simulink model "GS_model"  (R2018b)
settings: Solver=ode5  StartTime=0.0  StopTime=SimuStopTime  FixedStep=T_Simu  RelTol=1e-3
InitFcn:
  | Initial
undefined symbols (not defined in the file or in its folder): Aba10, Aba20, aeroCIP2006_S, aeroCIP2006_X, aeroCIP2006_Y, Agl0, Ass_kS, Ass_n1, Ass_n2, Ass_n3, Ass_n4, Ass_Noise, Ass_R, Ass_Resolution, Ass_TmOrder, AssA_Fix_Abs, AssB_Fix_Abs, AssC_Fix_Abs, AssD_Fix_Abs, AssE_Fix_Aps, AssF_Fix_Aps, C, c_max, c_min, Cd, CenterOfFigNX, CenterOfFigNY, CenterOfFigNZ, CenterOfFigP1, CenterOfFigP2, CenterOfFigPX, CenterOfFigPY, CenterOfFigPZ, Cmu, Crou, DEG2RAD, DiscIntNeverNeededParam, Eg_Dir, Eg_F, Eg_PrepareTime, Eg_r_L_L, Fw_Abf, Fw_Hmax, Fw_J, Fw_Spd0, Fw_Tmax, git_hash_BaseLine, git_hash_Project, Gnss_Noise_Pos, Gnss_Noise_Vel, Gnss_PropgationTime, GyroA_Fix_Abg, GyroA_Noise, GyroB_Fix_Abg, GyroB_Noise, GyroC_Fix_Abg, GyroC_Noise, GyroD_Fix_Abg, GyroD_Noise, h ... (+94)
libraries: simulink x308, sharedutil x46, aerolibutil x37, sharedtransform x31, vrlib x14, aerolibgravity2 x2
(part 12 of 20)

== system GS_model/Subsystem2/Subsystem/Sensor/Gyro/GyroBModel/GyroErrSet/GyroErrSet ==
  Wgi : Inport
  TC_GyroErrSet_Constant : Inport  Port=2
  TC_GyroErrSet_WildValue : Inport  Port=3
  TC_GyroErrSet_Jump : Inport  Port=4
  TC_StErrSet_Wave : Inport  Port=5
  GyroErrSet_Constant : Subsystem
  GyroErrSet_Jump : Subsystem
  GyroErrSet_Wave : Subsystem
  GyroErrSet_WildValue : Subsystem
  Wgi_g : Outport
  wires:
  GyroErrSet_WildValue/1(w_out) -> GyroErrSet_Jump/1(w_in)
  GyroErrSet_Constant/1(w_out) -> GyroErrSet_WildValue/1(w_in)
  GyroErrSet_Jump/1(w_out) -> GyroErrSet_Wave/1(w_in)
  Wgi/1 -> GyroErrSet_Constant/1(w_in)
  TC_GyroErrSet_Constant/1 -> GyroErrSet_Constant/2(ErrSwitch)
  TC_GyroErrSet_WildValue/1 -> GyroErrSet_WildValue/2(ErrSwitch)
  TC_GyroErrSet_Jump/1 -> GyroErrSet_Jump/2(ErrSet)
  TC_StErrSet_Wave/1 -> GyroErrSet_Wave/2(ErrSet)
  GyroErrSet_Wave/1(w_out) -> Wgi_g/1

== system GS_model/Subsystem2/Subsystem/Sensor/Gyro/GyroBModel/GyroErrSet/If Action Subsystem3 ==
  In1 : Inport
  Action Port : ActionPort  ActionType=else
  Out1 : Outport
  wires:
  In1/1 -> Out1/1

== system GS_model/Subsystem2/Subsystem/Sensor/Gyro/GyroBModel/GyroErrSet/If Action Subsystem4 ==
  In1 : Inport
  Action Port : ActionPort  ActionType=then
  Gain : Gain  Gain=DEG2RAD
  Out1 : Outport
  wires:
  In1/1 -> Gain/1
  Gain/1 -> Out1/1

== system GS_model/Subsystem2/Subsystem/Sensor/Gyro/GyroBModel/GyroErrSet/Triggered Subsystem5 ==
  In1 : Inport
  Enable : EnablePort
  Out1 : Outport  InitialOutput=0
  wires:
  In1/1 -> Out1/1

== system GS_model/Subsystem2/Subsystem/Sensor/Gyro/GyroBModel/GyroErrSet/Triggered Subsystem6 ==
  In1 : Inport
  Enable : EnablePort
  Out1 : Outport  InitialOutput=0
  wires:
  In1/1 -> Out1/1

== system GS_model/Subsystem2/Subsystem/Sensor/Gyro/GyroBModel/GyroErrSet/Triggered Subsystem7 ==
  In1 : Inport
  Enable : EnablePort
  Out1 : Outport
  wires:
  In1/1 -> Out1/1

== system GS_model/Subsystem2/Subsystem/Sensor/Gyro/GyroBModel/GyroErrSet/Triggered Subsystem8 ==
  In1 : Inport
  Enable : EnablePort
  Out1 : Outport
  wires:
  In1/1 -> Out1/1

== system GS_model/Subsystem2/Subsystem/Sensor/Gyro/GyroBModel/GyroErrSet/Triggered Subsystem9 ==
  In1 : Inport
  Enable : EnablePort
  Out1 : Outport
  wires:
  In1/1 -> Out1/1

== system GS_model/Subsystem2/Subsystem/Sensor/Gyro/GyroBModel/GyroMathModel/Triggered Subsystem1 ==
  In1 : Inport
  Enable : EnablePort
  Out1 : Outport  InitialOutput=0
  wires:
  In1/1 -> Out1/1

== system GS_model/Subsystem2/Subsystem/Sensor/Gyro/GyroCModel/GyroErrSet/GyroErrSet ==
  Wgi : Inport
  TC_GyroErrSet_Constant : Inport  Port=2
  TC_GyroErrSet_WildValue : Inport  Port=3
  TC_GyroErrSet_Jump : Inport  Port=4
  TC_StErrSet_Wave : Inport  Port=5
  GyroErrSet_Constant : Subsystem
  GyroErrSet_Jump : Subsystem
  GyroErrSet_Wave : Subsystem
  GyroErrSet_WildValue : Subsystem
  Wgi_g : Outport
  wires:
  GyroErrSet_WildValue/1(w_out) -> GyroErrSet_Jump/1(w_in)
  GyroErrSet_Constant/1(w_out) -> GyroErrSet_WildValue/1(w_in)
  GyroErrSet_Jump/1(w_out) -> GyroErrSet_Wave/1(w_in)
  Wgi/1 -> GyroErrSet_Constant/1(w_in)
  TC_GyroErrSet_Constant/1 -> GyroErrSet_Constant/2(ErrSwitch)
  TC_GyroErrSet_WildValue/1 -> GyroErrSet_WildValue/2(ErrSwitch)
  TC_GyroErrSet_Jump/1 -> GyroErrSet_Jump/2(ErrSet)
  TC_StErrSet_Wave/1 -> GyroErrSet_Wave/2(ErrSet)
  GyroErrSet_Wave/1(w_out) -> Wgi_g/1

== system GS_model/Subsystem2/Subsystem/Sensor/Gyro/GyroCModel/GyroErrSet/If Action Subsystem3 ==
  In1 : Inport
  Action Port : ActionPort  ActionType=else
  Out1 : Outport
  wires:
  In1/1 -> Out1/1

== system GS_model/Subsystem2/Subsystem/Sensor/Gyro/GyroCModel/GyroErrSet/If Action Subsystem4 ==
  In1 : Inport
  Action Port : ActionPort  ActionType=then
  Gain : Gain  Gain=DEG2RAD
  Out1 : Outport
  wires:
  In1/1 -> Gain/1
  Gain/1 -> Out1/1

== system GS_model/Subsystem2/Subsystem/Sensor/Gyro/GyroCModel/GyroErrSet/Triggered Subsystem5 ==
  In1 : Inport
  Enable : EnablePort
  Out1 : Outport  InitialOutput=0
  wires:
  In1/1 -> Out1/1

== system GS_model/Subsystem2/Subsystem/Sensor/Gyro/GyroCModel/GyroErrSet/Triggered Subsystem6 ==
  In1 : Inport
  Enable : EnablePort
  Out1 : Outport  InitialOutput=0
  wires:
  In1/1 -> Out1/1

== system GS_model/Subsystem2/Subsystem/Sensor/Gyro/GyroCModel/GyroErrSet/Triggered Subsystem7 ==
  In1 : Inport
  Enable : EnablePort
  Out1 : Outport
  wires:
  In1/1 -> Out1/1

== system GS_model/Subsystem2/Subsystem/Sensor/Gyro/GyroCModel/GyroErrSet/Triggered Subsystem8 ==
  In1 : Inport
  Enable : EnablePort
  Out1 : Outport
  wires:
  In1/1 -> Out1/1

== system GS_model/Subsystem2/Subsystem/Sensor/Gyro/GyroCModel/GyroErrSet/Triggered Subsystem9 ==
  In1 : Inport
  Enable : EnablePort
  Out1 : Outport
  wires:
  In1/1 -> Out1/1

== system GS_model/Subsystem2/Subsystem/Sensor/Gyro/GyroCModel/GyroMathModel/Triggered Subsystem1 ==
  In1 : Inport
  Enable : EnablePort
  Out1 : Outport  InitialOutput=0
  wires:
  In1/1 -> Out1/1

== system GS_model/Subsystem2/Subsystem/Sensor/Gyro/GyroDModel/GyroErrSet/GyroErrSet ==
  Wgi : Inport
  TC_GyroErrSet_Constant : Inport  Port=2
  TC_GyroErrSet_WildValue : Inport  Port=3
  TC_GyroErrSet_Jump : Inport  Port=4
  TC_StErrSet_Wave : Inport  Port=5
  GyroErrSet_Constant : Subsystem
  GyroErrSet_Jump : Subsystem
  GyroErrSet_Wave : Subsystem
  GyroErrSet_WildValue : Subsystem
  Wgi_g : Outport
  wires:
  GyroErrSet_WildValue/1(w_out) -> GyroErrSet_Jump/1(w_in)
  GyroErrSet_Constant/1(w_out) -> GyroErrSet_WildValue/1(w_in)
  GyroErrSet_Jump/1(w_out) -> GyroErrSet_Wave/1(w_in)
  Wgi/1 -> GyroErrSet_Constant/1(w_in)
  TC_GyroErrSet_Constant/1 -> GyroErrSet_Constant/2(ErrSwitch)
  TC_GyroErrSet_WildValue/1 -> GyroErrSet_WildValue/2(ErrSwitch)
  TC_GyroErrSet_Jump/1 -> GyroErrSet_Jump/2(ErrSet)
  TC_StErrSet_Wave/1 -> GyroErrSet_Wave/2(ErrSet)
  GyroErrSet_Wave/1(w_out) -> Wgi_g/1

== system GS_model/Subsystem2/Subsystem/Sensor/Gyro/GyroDModel/GyroErrSet/If Action Subsystem3 ==
  In1 : Inport
  Action Port : ActionPort  ActionType=else
  Out1 : Outport
  wires:
  In1/1 -> Out1/1

== system GS_model/Subsystem2/Subsystem/Sensor/Gyro/GyroDModel/GyroErrSet/If Action Subsystem4 ==
  In1 : Inport
  Action Port : ActionPort  ActionType=then
  Gain : Gain  Gain=DEG2RAD
  Out1 : Outport
  wires:
  In1/1 -> Gain/1
  Gain/1 -> Out1/1

== system GS_model/Subsystem2/Subsystem/Sensor/Gyro/GyroDModel/GyroErrSet/Triggered Subsystem5 ==
  In1 : Inport
  Enable : EnablePort
  Out1 : Outport  InitialOutput=0
  wires:
  In1/1 -> Out1/1

== system GS_model/Subsystem2/Subsystem/Sensor/Gyro/GyroDModel/GyroErrSet/Triggered Subsystem6 ==
  In1 : Inport
  Enable : EnablePort
  Out1 : Outport  InitialOutput=0
  wires:
  In1/1 -> Out1/1

== system GS_model/Subsystem2/Subsystem/Sensor/Gyro/GyroDModel/GyroErrSet/Triggered Subsystem7 ==
  In1 : Inport
  Enable : EnablePort
  Out1 : Outport
  wires:
  In1/1 -> Out1/1

== system GS_model/Subsystem2/Subsystem/Sensor/Gyro/GyroDModel/GyroErrSet/Triggered Subsystem8 ==
  In1 : Inport
  Enable : EnablePort
  Out1 : Outport
  wires:
  In1/1 -> Out1/1

== system GS_model/Subsystem2/Subsystem/Sensor/Gyro/GyroDModel/GyroErrSet/Triggered Subsystem9 ==
  In1 : Inport
  Enable : EnablePort
  Out1 : Outport
  wires:
  In1/1 -> Out1/1

== system GS_model/Subsystem2/Subsystem/Sensor/Gyro/GyroDModel/GyroMathModel/Triggered Subsystem1 ==
  In1 : Inport
  Enable : EnablePort
  Out1 : Outport  InitialOutput=0
  wires:
  In1/1 -> Out1/1

== system GS_model/Subsystem2/Subsystem/Sensor/Magnetometer/MmModel1/Mm_ErrSet/If Action Subsystem3 ==
  In1 : Inport
  Action Port : ActionPort  ActionType=else
  Out1 : Outport
  wires:
  In1/1 -> Out1/1

== system GS_model/Subsystem2/Subsystem/Sensor/Magnetometer/MmModel1/Mm_ErrSet/If Action Subsystem4 ==
  In1 : Inport
  Action Port : ActionPort  ActionType=then
  Out1 : Outport
  wires:
  In1/1 -> Out1/1

== system GS_model/Subsystem2/Subsystem/Sensor/Magnetometer/MmModel1/Mm_ErrSet/MmErrSet ==
  Mm_MagneticIntensity : Inport
  TC_MmErrSet_Constant : Inport  Port=2
  TC_MmErrSet_Jump : Inport  Port=3
  TC_MmErrSet_Wave : Inport  Port=4
  TC_MmErrSet_WildValue : Inport  Port=5
  MmErrSet_Constant : Subsystem
  MmErrSet_Jump : Subsystem
  MmErrSet_Wave : Subsystem
  MmErrSet_WildValue : Subsystem
  Mm_out : Outport
  wires:
  MmErrSet_WildValue/1(Mm_out) -> MmErrSet_Jump/1(Mm_in)
  MmErrSet_Constant/1(Mm_out) -> MmErrSet_WildValue/1(Mm_in)
  MmErrSet_Jump/1(Mm_out) -> MmErrSet_Wave/1(Mm_in)
  Mm_MagneticIntensity/1 -> MmErrSet_Constant/1(Mm_in)
  TC_MmErrSet_Constant/1 -> MmErrSet_Constant/2(ErrSwitch)
  TC_MmErrSet_WildValue/1 -> MmErrSet_WildValue/2(ErrSwitch)
  TC_MmErrSet_Jump/1 -> MmErrSet_Jump/2(ErrSet)
  TC_MmErrSet_Wave/1 -> MmErrSet_Wave/2(ErrSet)
  MmErrSet_Wave/1(Mm_out) -> Mm_out/1

== system GS_model/Subsystem2/Subsystem/Sensor/Magnetometer/MmModel1/Mm_ErrSet/Triggered Subsystem5 ==
  In1 : Inport
  Enable : EnablePort
  Out1 : Outport  InitialOutput=0
  wires:
  In1/1 -> Out1/1

== system GS_model/Subsystem2/Subsystem/Sensor/Magnetometer/MmModel1/Mm_ErrSet/Triggered Subsystem6 ==
  In1 : Inport
  Enable : EnablePort
  Out1 : Outport  InitialOutput=0
  wires:
  In1/1 -> Out1/1

== system GS_model/Subsystem2/Subsystem/Sensor/Magnetometer/MmModel1/Mm_ErrSet/Triggered Subsystem7 ==
  In1 : Inport
  Enable : EnablePort
  Out1 : Outport
  wires:
  In1/1 -> Out1/1

== system GS_model/Subsystem2/Subsystem/Sensor/Magnetometer/MmModel1/Mm_ErrSet/Triggered Subsystem8 ==
  In1 : Inport
  Enable : EnablePort
  Out1 : Outport
  wires:
  In1/1 -> Out1/1

== system GS_model/Subsystem2/Subsystem/Sensor/Magnetometer/MmModel1/Mm_ErrSet/Triggered Subsystem9 ==
  In1 : Inport
  Enable : EnablePort
  Out1 : Outport
  wires:
  In1/1 -> Out1/1

== system GS_model/Subsystem2/Subsystem/Sensor/Magnetometer/MmModel2/Mm_ErrSet/If Action Subsystem3 ==
  In1 : Inport
  Action Port : ActionPort  ActionType=else
  Out1 : Outport
  wires:
  In1/1 -> Out1/1

== system GS_model/Subsystem2/Subsystem/Sensor/Magnetometer/MmModel2/Mm_ErrSet/If Action Subsystem4 ==
  In1 : Inport
  Action Port : ActionPort  ActionType=then
  Out1 : Outport
  wires:
  In1/1 -> Out1/1

== system GS_model/Subsystem2/Subsystem/Sensor/Magnetometer/MmModel2/Mm_ErrSet/MmErrSet ==
  Mm_MagneticIntensity : Inport
  TC_MmErrSet_Constant : Inport  Port=2
  TC_MmErrSet_Jump : Inport  Port=3
  TC_MmErrSet_Wave : Inport  Port=4
  TC_MmErrSet_WildValue : Inport  Port=5
  MmErrSet_Constant : Subsystem
  MmErrSet_Jump : Subsystem
  MmErrSet_Wave : Subsystem
  MmErrSet_WildValue : Subsystem
  Mm_out : Outport
  wires:
  MmErrSet_Wave/1(Mm_out) -> Mm_out/1
  TC_MmErrSet_Wave/1 -> MmErrSet_Wave/2(ErrSet)
  TC_MmErrSet_Jump/1 -> MmErrSet_Jump/2(ErrSet)
  TC_MmErrSet_WildValue/1 -> MmErrSet_WildValue/2(ErrSwitch)
  TC_MmErrSet_Constant/1 -> MmErrSet_Constant/2(ErrSwitch)
  Mm_MagneticIntensity/1 -> MmErrSet_Constant/1(Mm_in)
  MmErrSet_Jump/1(Mm_out) -> MmErrSet_Wave/1(Mm_in)
  MmErrSet_Constant/1(Mm_out) -> MmErrSet_WildValue/1(Mm_in)
  MmErrSet_WildValue/1(Mm_out) -> MmErrSet_Jump/1(Mm_in)

== system GS_model/Subsystem2/Subsystem/Sensor/Magnetometer/MmModel2/Mm_ErrSet/Triggered Subsystem5 ==
  In1 : Inport
  Enable : EnablePort
  Out1 : Outport  InitialOutput=0
  wires:
  In1/1 -> Out1/1

== system GS_model/Subsystem2/Subsystem/Sensor/Magnetometer/MmModel2/Mm_ErrSet/Triggered Subsystem6 ==
  In1 : Inport
  Enable : EnablePort
  Out1 : Outport  InitialOutput=0
  wires:
  In1/1 -> Out1/1

== system GS_model/Subsystem2/Subsystem/Sensor/Magnetometer/MmModel2/Mm_ErrSet/Triggered Subsystem7 ==
  In1 : Inport
  Enable : EnablePort
  Out1 : Outport
  wires:
  In1/1 -> Out1/1

== system GS_model/Subsystem2/Subsystem/Sensor/Magnetometer/MmModel2/Mm_ErrSet/Triggered Subsystem8 ==
  In1 : Inport
  Enable : EnablePort
  Out1 : Outport
  wires:
  In1/1 -> Out1/1

== system GS_model/Subsystem2/Subsystem/Sensor/Magnetometer/MmModel2/Mm_ErrSet/Triggered Subsystem9 ==
  In1 : Inport
  Enable : EnablePort
  Out1 : Outport
  wires:
  In1/1 -> Out1/1

== system GS_model/Subsystem2/Subsystem/Sensor/Magnetometer/MmModel3/Mm_ErrSet/If Action Subsystem3 ==
  In1 : Inport
  Action Port : ActionPort  ActionType=else
  Out1 : Outport
  wires:
  In1/1 -> Out1/1

== system GS_model/Subsystem2/Subsystem/Sensor/Magnetometer/MmModel3/Mm_ErrSet/If Action Subsystem4 ==
  In1 : Inport
  Action Port : ActionPort  ActionType=then
  Out1 : Outport
  wires:
  In1/1 -> Out1/1

== system GS_model/Subsystem2/Subsystem/Sensor/Magnetometer/MmModel3/Mm_ErrSet/MmErrSet ==
  Mm_MagneticIntensity : Inport
  TC_MmErrSet_Constant : Inport  Port=2
  TC_MmErrSet_Jump : Inport  Port=3
  TC_MmErrSet_Wave : Inport  Port=4
  TC_MmErrSet_WildValue : Inport  Port=5
  MmErrSet_Constant : Subsystem
  MmErrSet_Jump : Subsystem
  MmErrSet_Wave : Subsystem
  MmErrSet_WildValue : Subsystem
  Mm_out : Outport
  wires:
  MmErrSet_WildValue/1(Mm_out) -> MmErrSet_Jump/1(Mm_in)
  MmErrSet_Constant/1(Mm_out) -> MmErrSet_WildValue/1(Mm_in)
  MmErrSet_Jump/1(Mm_out) -> MmErrSet_Wave/1(Mm_in)
  Mm_MagneticIntensity/1 -> MmErrSet_Constant/1(Mm_in)
  TC_MmErrSet_Constant/1 -> MmErrSet_Constant/2(ErrSwitch)
  TC_MmErrSet_WildValue/1 -> MmErrSet_WildValue/2(ErrSwitch)
  TC_MmErrSet_Jump/1 -> MmErrSet_Jump/2(ErrSet)
  TC_MmErrSet_Wave/1 -> MmErrSet_Wave/2(ErrSet)
  MmErrSet_Wave/1(Mm_out) -> Mm_out/1

== system GS_model/Subsystem2/Subsystem/Sensor/Magnetometer/MmModel3/Mm_ErrSet/Triggered Subsystem5 ==
  In1 : Inport
  Enable : EnablePort
  Out1 : Outport  InitialOutput=0
  wires:
  In1/1 -> Out1/1

== system GS_model/Subsystem2/Subsystem/Sensor/Magnetometer/MmModel3/Mm_ErrSet/Triggered Subsystem6 ==
  In1 : Inport
  Enable : EnablePort
  Out1 : Outport  InitialOutput=0
  wires:
  In1/1 -> Out1/1

== system GS_model/Subsystem2/Subsystem/Sensor/Magnetometer/MmModel3/Mm_ErrSet/Triggered Subsystem7 ==
  In1 : Inport
  Enable : EnablePort
  Out1 : Outport
  wires:
  In1/1 -> Out1/1

== system GS_model/Subsystem2/Subsystem/Sensor/Magnetometer/MmModel3/Mm_ErrSet/Triggered Subsystem8 ==
  In1 : Inport
  Enable : EnablePort
  Out1 : Outport
  wires:
  In1/1 -> Out1/1

== system GS_model/Subsystem2/Subsystem/Sensor/Magnetometer/MmModel3/Mm_ErrSet/Triggered Subsystem9 ==
  In1 : Inport
  Enable : EnablePort
  Out1 : Outport
  wires:
  In1/1 -> Out1/1

== system GS_model/Subsystem2/Subsystem/Sensor/Magnetometer/MmModel4/Mm_ErrSet/If Action Subsystem3 ==
  In1 : Inport
  Action Port : ActionPort  ActionType=else
  Out1 : Outport
  wires:
  In1/1 -> Out1/1

== system GS_model/Subsystem2/Subsystem/Sensor/Magnetometer/MmModel4/Mm_ErrSet/If Action Subsystem4 ==
  In1 : Inport
  Action Port : ActionPort  ActionType=then
  Out1 : Outport
  wires:
  In1/1 -> Out1/1

== system GS_model/Subsystem2/Subsystem/Sensor/Magnetometer/MmModel4/Mm_ErrSet/MmErrSet ==
  Mm_MagneticIntensity : Inport
  TC_MmErrSet_Constant : Inport  Port=2
  TC_MmErrSet_Jump : Inport  Port=3
  TC_MmErrSet_Wave : Inport  Port=4
  TC_MmErrSet_WildValue : Inport  Port=5
  MmErrSet_Constant : Subsystem
  MmErrSet_Jump : Subsystem
  MmErrSet_Wave : Subsystem
  MmErrSet_WildValue : Subsystem
  Mm_out : Outport
  wires:
  MmErrSet_Wave/1(Mm_out) -> Mm_out/1
  TC_MmErrSet_Wave/1 -> MmErrSet_Wave/2(ErrSet)
  TC_MmErrSet_Jump/1 -> MmErrSet_Jump/2(ErrSet)
  TC_MmErrSet_WildValue/1 -> MmErrSet_WildValue/2(ErrSwitch)
  TC_MmErrSet_Constant/1 -> MmErrSet_Constant/2(ErrSwitch)
  Mm_MagneticIntensity/1 -> MmErrSet_Constant/1(Mm_in)
  MmErrSet_Jump/1(Mm_out) -> MmErrSet_Wave/1(Mm_in)
  MmErrSet_Constant/1(Mm_out) -> MmErrSet_WildValue/1(Mm_in)
  MmErrSet_WildValue/1(Mm_out) -> MmErrSet_Jump/1(Mm_in)

== system GS_model/Subsystem2/Subsystem/Sensor/Magnetometer/MmModel4/Mm_ErrSet/Triggered Subsystem5 ==
  In1 : Inport
  Enable : EnablePort
  Out1 : Outport  InitialOutput=0
  wires:
  In1/1 -> Out1/1

== system GS_model/Subsystem2/Subsystem/Sensor/Magnetometer/MmModel4/Mm_ErrSet/Triggered Subsystem6 ==
  In1 : Inport
  Enable : EnablePort
  Out1 : Outport  InitialOutput=0
  wires:
  In1/1 -> Out1/1

== system GS_model/Subsystem2/Subsystem/Sensor/Magnetometer/MmModel4/Mm_ErrSet/Triggered Subsystem7 ==
  In1 : Inport
  Enable : EnablePort
  Out1 : Outport
  wires:
  In1/1 -> Out1/1

== system GS_model/Subsystem2/Subsystem/Sensor/Magnetometer/MmModel4/Mm_ErrSet/Triggered Subsystem8 ==
  In1 : Inport
  Enable : EnablePort
  Out1 : Outport
  wires:
  In1/1 -> Out1/1

== system GS_model/Subsystem2/Subsystem/Sensor/Magnetometer/MmModel4/Mm_ErrSet/Triggered Subsystem9 ==
  In1 : Inport
  Enable : EnablePort
  Out1 : Outport
  wires:
  In1/1 -> Out1/1

== system GS_model/Subsystem2/Subsystem/Sensor/StA&B&C&DModel1/StAMathModel/StErrSet/From Q to W ==
  q : Inport
  Acos : Trigonometry  Operator=acos
  Delay : Delay  DelayLength=1
  Demux6 : Demux  Outputs=[1;3]
  Gain : Gain  Gain=2/T_Simu
  Normalize Vector : vrlib/Utilities/Normalize Vector  maxzero=0
  Product : Product
  Product1 : Product
  Quaternion Division : aerolibutil/Quaternion Division
      settings: SourceProductBaseCode=AE
  Selector : Selector  InputPortWidth=4  IndexOptions=Index vector (dialog)  Indices=1  OutputSizes=1
  Sign : Signum
  w : Outport
  wires:
  Acos/1 -> Gain/1
  Demux6/1 -> Acos/1
  Gain/1 -> Product/1
  q/1 -> Delay/1, Quaternion Division/1
  Demux6/2 -> Normalize Vector/1
  Product/1 -> w/1
  Normalize Vector/1 -> Product/2
  Delay/1 -> Quaternion Division/2
  Selector/1 -> Sign/1
  Quaternion Division/1 -> Selector/1, Product1/2
  Sign/1 -> Product1/1
  Product1/1 -> Demux6/1

== system GS_model/Subsystem2/Subsystem/Sensor/StA&B&C&DModel1/StAMathModel/StErrSet/If Action Subsystem ==
  In1 : Inport
  Action Port : ActionPort  ActionType=then
  Out1 : Outport
  wires:
  In1/1 -> Out1/1

== system GS_model/Subsystem2/Subsystem/Sensor/StA&B&C&DModel1/StAMathModel/StErrSet/If Action Subsystem1 ==
  In1 : Inport
  Action Port : ActionPort  ActionType=else
  Out1 : Outport
  wires:
  In1/1 -> Out1/1

== system GS_model/Subsystem2/Subsystem/Sensor/StA&B&C&DModel1/StAMathModel/StErrSet/StAErrSet ==
  note: Switch
  note: Period
  note: AmpCoff
  note: Switch
  note: Amp
  Qis_St : Inport
  TC_StErr_Constant : Inport  Port=2
  TC_StErr_WildValue : Inport  Port=3
  TC_StErr_Jump : Inport  Port=4
  TC_StErr_Wave : Inport  Port=5
  AssErrSet_WildValue : Subsystem
  Demux : Demux  Outputs=2
  Demux1 : Demux  Outputs=3
  JumpSet : Constant  Value=[0;6/180*pi;0]
  StErrSet_Constant : Subsystem
  StErrSet_Jump : Subsystem
  StErrSet_Wave : Subsystem
  Terminator : Terminator
  WaveSet : SignalGenerator  WaveForm=square  Amplitude=1/180*pi
  WildValueSet : Constant  Value=1.2
  TM_St_Qis : Outport
  wires:
  TC_StErr_Wave/1 -> Demux/1
  Qis_St/1 -> StErrSet_Constant/1(Q_in)
  TC_StErr_Constant/1 -> StErrSet_Constant/2(ErrSwitch)
  StErrSet_Constant/1(Q_out) -> AssErrSet_WildValue/1(Qin)
  TC_StErr_WildValue/1 -> AssErrSet_WildValue/3(ErrSwitch)
  WildValueSet/1 -> AssErrSet_WildValue/2(ErrValue)
  AssErrSet_WildValue/1(Q_out) -> StErrSet_Jump/1(Qin)
  JumpSet/1 -> StErrSet_Jump/2(ErrValue)
  Demux1/2 -> Terminator/1
  TC_StErr_Jump/1 -> Demux1/1
  Demux1/1 -> StErrSet_Jump/3(ErrSwitch)
  Demux1/3 -> StErrSet_Jump/4(StJumpErrAmpCoff)
  StErrSet_Jump/1(Q_out) -> StErrSet_Wave/1(Qin)
  StErrSet_Wave/1(Q_out) -> TM_St_Qis/1
  WaveSet/1 -> StErrSet_Wave/2(ErrValue)
  Demux/1 -> StErrSet_Wave/3(ErrSwitch)
  Demux/2 -> StErrSet_Wave/4(StWaveErrAmp)

== system GS_model/Subsystem2/Subsystem/Sensor/StA&B&C&DModel1/StAMathModel/StErrSet/Triggered Subsystem1 ==
  In1 : Inport
  Enable : EnablePort
  Out1 : Outport  InitialOutput=0
  wires:
  In1/1 -> Out1/1

== system GS_model/Subsystem2/Subsystem/Sensor/StA&B&C&DModel1/StAMathModel/StErrSet/Triggered Subsystem2 ==
  In1 : Inport
  Enable : EnablePort
  Out1 : Outport
  wires:
  In1/1 -> Out1/1

== system GS_model/Subsystem2/Subsystem/Sensor/StA&B&C&DModel1/StAMathModel/StErrSet/Triggered Subsystem3 ==
  In1 : Inport
  Enable : EnablePort
  Out1 : Outport
  wires:
  In1/1 -> Out1/1

== system GS_model/Subsystem2/Subsystem/Sensor/StA&B&C&DModel1/StAMathModel/StErrSet/Triggered Subsystem4 ==
  In1 : Inport
  Enable : EnablePort
  Out1 : Outport
  wires:
  In1/1 -> Out1/1

== system GS_model/Subsystem2/Subsystem/Sensor/StA&B&C&DModel1/StAMathModel/StErrSet/Triggered Subsystem5 ==
  In1 : Inport
  Enable : EnablePort
  Out1 : Outport  InitialOutput=0
  wires:
  In1/1 -> Out1/1

== system GS_model/Subsystem2/Subsystem/Sensor/StA&B&C&DModel1/StAMathModel/StMathModel/3 ==
  TC_StNoiseCoff : Inport
  Cons_StNoise : Inport  Port=2
  Constant : Constant
  Demux : Demux
  Mux : Mux  Inputs=2
  Product : Product
  Quaternion Normalize : sharedutil/Quaternion Normalize  aMode=aMode
      settings: SourceProductBaseCode=AE,PW,MT,VE,VP
  VoltA1 : Scope  NumInputPorts=4
  theta/2 : Gain  Gain=0.5
  Q_StNoise : Outport
  wires:
  Mux/1 -> Quaternion Normalize/1, Demux/1
  Quaternion Normalize/1 -> Q_StNoise/1
  Constant/1 -> Mux/1
  Demux/2 -> VoltA1/2
  Demux/3 -> VoltA1/3
  Demux/4 -> VoltA1/4
  Demux/1 -> VoltA1/1
  Cons_StNoise/1 -> Product/1
  TC_StNoiseCoff/1 -> Product/2
  Product/1 -> theta/2/1
  theta/2/1 -> Mux/2

== system GS_model/Subsystem2/Subsystem/Sensor/StA&B&C&DModel1/StAMathModel/StMathModel/Triggered Subsystem1 ==
  In1 : Inport
  Enable : EnablePort
  Out1 : Outport  InitialOutput=[1;0;0;0]
  wires:
  In1/1 -> Out1/1

== system GS_model/Subsystem2/Subsystem/Sensor/StA&B&C&DModel1/StAMathModel/StMathModel/Triggered Subsystem2 ==
  In1 : Inport
  Enable : EnablePort
  Out1 : Outport  InitialOutput=1
  wires:
  In1/1 -> Out1/1

== system GS_model/Subsystem2/Subsystem/Sensor/StA&B&C&DModel1/StAMathModel/Subsystem/Subsystem ==
  note: Qbs
  Sun_b : Inport
  Sunshine : Inport  Port=2
  Qsb_StAFix : Inport  Port=3
  SEA : Inport  Port=4
  EEA : Inport  Port=5
  Qob : Inport  Port=6
  Acos : Trigonometry  Operator=acos
  Acos1 : Trigonometry  Operator=acos
  Compare To Constant : simulink/Logic and Bit Operations/Compare To Constant  relop===  const=1  OutDataTypeStr=boolean
  Constant : Constant  Value=St_SightAxis
  Constant1 : Constant  Value=[0;0;1]
  Constant3 : Constant  Value=St_EarthAtomAgl
  Cos : Trigonometry  Operator=cos
  Cos1 : Trigonometry  Operator=cos
  Data Type Conversion : DataTypeConversion  OutDataTypeStr=double
  Logical Operator : Logic  AllPortsSameDT=off  OutDataTypeStr=boolean
  Logical Operator1 : Logic  Operator=OR  AllPortsSameDT=off  OutDataTypeStr=boolean
  Logical Operator2 : Logic  Operator=NOT  AllPortsSameDT=off  OutDataTypeStr=boolean
  MatrixMultiply{,1..4} (5 alike) : Product  Multiplication=Matrix(*)
  Mux : Mux  Inputs=2
  Quaternion Inverse : aerolibutil/Quaternion Inverse
  Quaternions to Direction Cosine Matrix : sharedtransform/Quaternions to  Direction Cosine Matrix  aMode=aMode
      settings: SourceProductBaseCode=AE,PW,MT,VE,VP
  Quaternions to Direction Cosine Matrix1 : sharedtransform/Quaternions to  Direction Cosine Matrix  aMode=aMode
      settings: SourceProductBaseCode=AE,PW,MT,VE,VP
  Relational Operator : RelationalOperator  OutDataTypeStr=boolean  RndMeth=Simplest
  Relational Operator1 : RelationalOperator  OutDataTypeStr=boolean  RndMeth=Simplest
  Sum : Sum  Inputs=|++
  Transpose : Math  Operator=transpose  SaturateOnIntegerOverflow=on
  Valid : Outport
  Agl_St&SunEarth : Outport  Port=2
  wires:
  Transpose/1 -> MatrixMultiply4/1, MatrixMultiply1/1
  Constant3/1 -> Sum/2
  Logical Operator/1 -> Logical Operator1/1
  Cos/1 -> Relational Operator/2
  Quaternions to Direction Cosine Matrix1/1 -> MatrixMultiply2/1
  SEA/1 -> Cos/1
  Qob/1 -> Quaternions to Direction Cosine Matrix1/1
  MatrixMultiply3/1 -> MatrixMultiply4/2
  Qsb_StAFix/1 -> Quaternion Inverse/1
  Quaternions to Direction Cosine Matrix/1 -> MatrixMultiply3/1, MatrixMultiply/1
  Sun_b/1 -> MatrixMultiply/2
  Constant1/1 -> MatrixMultiply2/2
  MatrixMultiply2/1 -> MatrixMultiply3/2
  Cos1/1 -> Relational Operator1/2
  Quaternion Inverse/1 -> Quaternions to Direction Cosine Matrix/1
  Relational Operator/1 -> Logical Operator/2
  Constant/1 -> Transpose/1
  MatrixMultiply4/1 -> Acos1/1, Relational Operator1/1
  Sunshine/1 -> Compare To Constant/1
  EEA/1 -> Sum/1
  Relational Operator1/1 -> Logical Operator1/2
  Acos/1 -> Mux/1
  Acos1/1 -> Mux/2
  Sum/1 -> Cos1/1
  MatrixMultiply1/1 -> Relational Operator/1, Acos/1
  Compare To Constant/1 -> Logical Operator/1
  MatrixMultiply/1 -> MatrixMultiply1/2
  Mux/1 -> Agl_St&SunEarth/1
  Logical Operator2/1 -> Data Type Conversion/1
  Data Type Conversion/1 -> Valid/1
  Logical Operator1/1 -> Logical Operator2/1

== system GS_model/Subsystem2/Subsystem/Sensor/StA&B&C&DModel1/StAMathModel/Subsystem/Triggered Subsystem2 ==
  In1 : Inport
  Enable : EnablePort
  Out1 : Outport  InitialOutput=1
  wires:
  In1/1 -> Out1/1

== system GS_model/Subsystem2/Subsystem/Sensor/StA&B&C&DModel1/StAMathModel1/StErrSet/From Q to W ==
  q : Inport
  Acos : Trigonometry  Operator=acos
  Delay : Delay  DelayLength=1
  Demux6 : Demux  Outputs=[1;3]
  Gain : Gain  Gain=2/T_Simu
  Normalize Vector : vrlib/Utilities/Normalize Vector  maxzero=0
  Product : Product
  Product1 : Product
  Quaternion Division : aerolibutil/Quaternion Division
      settings: SourceProductBaseCode=AE
  Selector : Selector  InputPortWidth=4  IndexOptions=Index vector (dialog)  Indices=1  OutputSizes=1
  Sign : Signum
  w : Outport
  wires:
  Product1/1 -> Demux6/1
  Sign/1 -> Product1/1
  Quaternion Division/1 -> Product1/2, Selector/1
  Selector/1 -> Sign/1
  Delay/1 -> Quaternion Division/2
  Normalize Vector/1 -> Product/2
  Product/1 -> w/1
  Demux6/2 -> Normalize Vector/1
  q/1 -> Quaternion Division/1, Delay/1
  Gain/1 -> Product/1
  Demux6/1 -> Acos/1
  Acos/1 -> Gain/1

== system GS_model/Subsystem2/Subsystem/Sensor/StA&B&C&DModel1/StAMathModel1/StErrSet/If Action Subsystem ==
  In1 : Inport
  Action Port : ActionPort  ActionType=then
  Out1 : Outport
  wires:
  In1/1 -> Out1/1

== system GS_model/Subsystem2/Subsystem/Sensor/StA&B&C&DModel1/StAMathModel1/StErrSet/If Action Subsystem1 ==
  In1 : Inport
  Action Port : ActionPort  ActionType=else
  Out1 : Outport
  wires:
  In1/1 -> Out1/1

== system GS_model/Subsystem2/Subsystem/Sensor/StA&B&C&DModel1/StAMathModel1/StErrSet/StAErrSet ==
  note: Amp
  note: Switch
  note: AmpCoff
  note: Period
  note: Switch
  Qis_St : Inport
  TC_StErr_Constant : Inport  Port=2
  TC_StErr_WildValue : Inport  Port=3
  TC_StErr_Jump : Inport  Port=4
  TC_StErr_Wave : Inport  Port=5
  AssErrSet_WildValue : Subsystem
  Demux : Demux  Outputs=2
  Demux1 : Demux  Outputs=3
  JumpSet : Constant  Value=[0;6/180*pi;0]
  StErrSet_Constant : Subsystem
  StErrSet_Jump : Subsystem
  StErrSet_Wave : Subsystem
  Terminator : Terminator
  WaveSet : SignalGenerator  WaveForm=square  Amplitude=1/180*pi
  WildValueSet : Constant  Value=1.2
  TM_St_Qis : Outport
  wires:
  Demux/2 -> StErrSet_Wave/4(StWaveErrAmp)
  Demux/1 -> StErrSet_Wave/3(ErrSwitch)
  WaveSet/1 -> StErrSet_Wave/2(ErrValue)
  StErrSet_Wave/1(Q_out) -> TM_St_Qis/1
  StErrSet_Jump/1(Q_out) -> StErrSet_Wave/1(Qin)
  Demux1/3 -> StErrSet_Jump/4(StJumpErrAmpCoff)
  Demux1/1 -> StErrSet_Jump/3(ErrSwitch)
  TC_StErr_Jump/1 -> Demux1/1
  Demux1/2 -> Terminator/1
  JumpSet/1 -> StErrSet_Jump/2(ErrValue)
  AssErrSet_WildValue/1(Q_out) -> StErrSet_Jump/1(Qin)
  WildValueSet/1 -> AssErrSet_WildValue/2(ErrValue)
  TC_StErr_WildValue/1 -> AssErrSet_WildValue/3(ErrSwitch)
  StErrSet_Constant/1(Q_out) -> AssErrSet_WildValue/1(Qin)
  TC_StErr_Constant/1 -> StErrSet_Constant/2(ErrSwitch)
  Qis_St/1 -> StErrSet_Constant/1(Q_in)
  TC_StErr_Wave/1 -> Demux/1

== system GS_model/Subsystem2/Subsystem/Sensor/StA&B&C&DModel1/StAMathModel1/StErrSet/Triggered Subsystem1 ==
  In1 : Inport
  Enable : EnablePort
  Out1 : Outport  InitialOutput=0
  wires:
  In1/1 -> Out1/1

== system GS_model/Subsystem2/Subsystem/Sensor/StA&B&C&DModel1/StAMathModel1/StErrSet/Triggered Subsystem2 ==
  In1 : Inport
  Enable : EnablePort
  Out1 : Outport
  wires:
  In1/1 -> Out1/1

== system GS_model/Subsystem2/Subsystem/Sensor/StA&B&C&DModel1/StAMathModel1/StErrSet/Triggered Subsystem3 ==
  In1 : Inport
  Enable : EnablePort
  Out1 : Outport
  wires:
  In1/1 -> Out1/1

== system GS_model/Subsystem2/Subsystem/Sensor/StA&B&C&DModel1/StAMathModel1/StErrSet/Triggered Subsystem4 ==
  In1 : Inport
  Enable : EnablePort
  Out1 : Outport
  wires:
  In1/1 -> Out1/1

== system GS_model/Subsystem2/Subsystem/Sensor/StA&B&C&DModel1/StAMathModel1/StErrSet/Triggered Subsystem5 ==
  In1 : Inport
  Enable : EnablePort
  Out1 : Outport  InitialOutput=0
  wires:
  In1/1 -> Out1/1

== system GS_model/Subsystem2/Subsystem/Sensor/StA&B&C&DModel1/StAMathModel1/StMathModel/3 ==
  TC_StNoiseCoff : Inport
  Cons_StNoise : Inport  Port=2
  Constant : Constant
  Demux : Demux
  Mux : Mux  Inputs=2
  Product : Product
  Quaternion Normalize : sharedutil/Quaternion Normalize  aMode=aMode
      settings: SourceProductBaseCode=AE,PW,MT,VE,VP
  VoltA1 : Scope  NumInputPorts=4
  theta/2 : Gain  Gain=0.5
  Q_StNoise : Outport
  wires:
  theta/2/1 -> Mux/2
  Product/1 -> theta/2/1
  TC_StNoiseCoff/1 -> Product/2
  Cons_StNoise/1 -> Product/1
  Demux/1 -> VoltA1/1
  Demux/4 -> VoltA1/4
  Demux/3 -> VoltA1/3
  Demux/2 -> VoltA1/2
  Constant/1 -> Mux/1
  Quaternion Normalize/1 -> Q_StNoise/1
  Mux/1 -> Demux/1, Quaternion Normalize/1

== system GS_model/Subsystem2/Subsystem/Sensor/StA&B&C&DModel1/StAMathModel1/StMathModel/Triggered Subsystem1 ==
  In1 : Inport
  Enable : EnablePort
  Out1 : Outport  InitialOutput=[1;0;0;0]
  wires:
  In1/1 -> Out1/1

== system GS_model/Subsystem2/Subsystem/Sensor/StA&B&C&DModel1/StAMathModel1/StMathModel/Triggered Subsystem2 ==
  In1 : Inport
  Enable : EnablePort
  Out1 : Outport  InitialOutput=1
  wires:
  In1/1 -> Out1/1

== system GS_model/Subsystem2/Subsystem/Sensor/StA&B&C&DModel1/StAMathModel1/Subsystem/Subsystem ==
  note: Qbs
  Sun_b : Inport
  Sunshine : Inport  Port=2
  Qsb_StAFix : Inport  Port=3
  SEA : Inport  Port=4
  EEA : Inport  Port=5
  Qob : Inport  Port=6
  Acos : Trigonometry  Operator=acos
  Acos1 : Trigonometry  Operator=acos
  Compare To Constant : simulink/Logic and Bit Operations/Compare To Constant  relop===  const=1  OutDataTypeStr=boolean
  Constant : Constant  Value=St_SightAxis
  Constant1 : Constant  Value=[0;0;1]
  Constant3 : Constant  Value=St_EarthAtomAgl
  Cos : Trigonometry  Operator=cos
  Cos1 : Trigonometry  Operator=cos
  Data Type Conversion : DataTypeConversion  OutDataTypeStr=double
  Logical Operator : Logic  AllPortsSameDT=off  OutDataTypeStr=boolean
  Logical Operator1 : Logic  Operator=OR  AllPortsSameDT=off  OutDataTypeStr=boolean
  Logical Operator2 : Logic  Operator=NOT  AllPortsSameDT=off  OutDataTypeStr=boolean
  MatrixMultiply{,1..4} (5 alike) : Product  Multiplication=Matrix(*)
  Mux : Mux  Inputs=2
  Quaternion Inverse : aerolibutil/Quaternion Inverse
  Quaternions to Direction Cosine Matrix : sharedtransform/Quaternions to  Direction Cosine Matrix  aMode=aMode
      settings: SourceProductBaseCode=AE,PW,MT,VE,VP
  Quaternions to Direction Cosine Matrix1 : sharedtransform/Quaternions to  Direction Cosine Matrix  aMode=aMode
      settings: SourceProductBaseCode=AE,PW,MT,VE,VP
  Relational Operator : RelationalOperator  OutDataTypeStr=boolean  RndMeth=Simplest
  Relational Operator1 : RelationalOperator  OutDataTypeStr=boolean  RndMeth=Simplest
  Sum : Sum  Inputs=|++
  Transpose : Math  Operator=transpose  SaturateOnIntegerOverflow=on
  Valid : Outport
  Agl_St&SunEarth : Outport  Port=2
  wires:
  Logical Operator1/1 -> Logical Operator2/1
  Data Type Conversion/1 -> Valid/1
  Logical Operator2/1 -> Data Type Conversion/1
  Mux/1 -> Agl_St&SunEarth/1
  MatrixMultiply/1 -> MatrixMultiply1/2
  Compare To Constant/1 -> Logical Operator/1
  MatrixMultiply1/1 -> Acos/1, Relational Operator/1
  Sum/1 -> Cos1/1
  Acos1/1 -> Mux/2
  Acos/1 -> Mux/1
  Relational Operator1/1 -> Logical Operator1/2
  EEA/1 -> Sum/1
  Sunshine/1 -> Compare To Constant/1
  MatrixMultiply4/1 -> Relational Operator1/1, Acos1/1
  Constant/1 -> Transpose/1
  Relational Operator/1 -> Logical Operator/2
  Quaternion Inverse/1 -> Quaternions to Direction Cosine Matrix/1
  Cos1/1 -> Relational Operator1/2
  MatrixMultiply2/1 -> MatrixMultiply3/2
  Constant1/1 -> MatrixMultiply2/2
  Sun_b/1 -> MatrixMultiply/2
  Quaternions to Direction Cosine Matrix/1 -> MatrixMultiply/1, MatrixMultiply3/1
  Qsb_StAFix/1 -> Quaternion Inverse/1
  MatrixMultiply3/1 -> MatrixMultiply4/2
  Qob/1 -> Quaternions to Direction Cosine Matrix1/1
  SEA/1 -> Cos/1
  Quaternions to Direction Cosine Matrix1/1 -> MatrixMultiply2/1
  Cos/1 -> Relational Operator/2
  Logical Operator/1 -> Logical Operator1/1
  Constant3/1 -> Sum/2
  Transpose/1 -> MatrixMultiply1/1, MatrixMultiply4/1

== system GS_model/Subsystem2/Subsystem/Sensor/StA&B&C&DModel1/StAMathModel1/Subsystem/Triggered Subsystem2 ==
  In1 : Inport
  Enable : EnablePort
  Out1 : Outport  InitialOutput=1
  wires:
  In1/1 -> Out1/1

== system GS_model/Subsystem2/Subsystem/Sensor/StA&B&C&DModel1/StAMathModel2/StErrSet/From Q to W ==
  q : Inport
  Acos : Trigonometry  Operator=acos
  Delay : Delay  DelayLength=1
  Demux6 : Demux  Outputs=[1;3]
  Gain : Gain  Gain=2/T_Simu
  Normalize Vector : vrlib/Utilities/Normalize Vector  maxzero=0
  Product : Product
  Product1 : Product
  Quaternion Division : aerolibutil/Quaternion Division
      settings: SourceProductBaseCode=AE
  Selector : Selector  InputPortWidth=4  IndexOptions=Index vector (dialog)  Indices=1  OutputSizes=1
  Sign : Signum
  w : Outport
  wires:
  Acos/1 -> Gain/1
  Demux6/1 -> Acos/1
  Gain/1 -> Product/1
  q/1 -> Delay/1, Quaternion Division/1
  Demux6/2 -> Normalize Vector/1
  Product/1 -> w/1
  Normalize Vector/1 -> Product/2
  Delay/1 -> Quaternion Division/2
  Selector/1 -> Sign/1
  Quaternion Division/1 -> Selector/1, Product1/2
  Sign/1 -> Product1/1
  Product1/1 -> Demux6/1

== system GS_model/Subsystem2/Subsystem/Sensor/StA&B&C&DModel1/StAMathModel2/StErrSet/If Action Subsystem ==
  In1 : Inport
  Action Port : ActionPort  ActionType=then
  Out1 : Outport
  wires:
  In1/1 -> Out1/1

== system GS_model/Subsystem2/Subsystem/Sensor/StA&B&C&DModel1/StAMathModel2/StErrSet/If Action Subsystem1 ==
  In1 : Inport
  Action Port : ActionPort  ActionType=else
  Out1 : Outport
  wires:
  In1/1 -> Out1/1

== system GS_model/Subsystem2/Subsystem/Sensor/StA&B&C&DModel1/StAMathModel2/StErrSet/StAErrSet ==
  note: Switch
  note: Period
  note: AmpCoff
  note: Switch
  note: Amp
  Qis_St : Inport
  TC_StErr_Constant : Inport  Port=2
  TC_StErr_WildValue : Inport  Port=3
  TC_StErr_Jump : Inport  Port=4
  TC_StErr_Wave : Inport  Port=5
  AssErrSet_WildValue : Subsystem
  Demux : Demux  Outputs=2
  Demux1 : Demux  Outputs=3
  JumpSet : Constant  Value=[0;6/180*pi;0]
  StErrSet_Constant : Subsystem
  StErrSet_Jump : Subsystem
  StErrSet_Wave : Subsystem
  Terminator : Terminator
  WaveSet : SignalGenerator  WaveForm=square  Amplitude=1/180*pi
  WildValueSet : Constant  Value=1.2
  TM_St_Qis : Outport
  wires:
  TC_StErr_Wave/1 -> Demux/1
  Qis_St/1 -> StErrSet_Constant/1(Q_in)
  TC_StErr_Constant/1 -> StErrSet_Constant/2(ErrSwitch)
  StErrSet_Constant/1(Q_out) -> AssErrSet_WildValue/1(Qin)
  TC_StErr_WildValue/1 -> AssErrSet_WildValue/3(ErrSwitch)
  WildValueSet/1 -> AssErrSet_WildValue/2(ErrValue)
  AssErrSet_WildValue/1(Q_out) -> StErrSet_Jump/1(Qin)
  JumpSet/1 -> StErrSet_Jump/2(ErrValue)
  Demux1/2 -> Terminator/1
  TC_StErr_Jump/1 -> Demux1/1
  Demux1/1 -> StErrSet_Jump/3(ErrSwitch)
  Demux1/3 -> StErrSet_Jump/4(StJumpErrAmpCoff)
  StErrSet_Jump/1(Q_out) -> StErrSet_Wave/1(Qin)
  StErrSet_Wave/1(Q_out) -> TM_St_Qis/1
  WaveSet/1 -> StErrSet_Wave/2(ErrValue)
  Demux/1 -> StErrSet_Wave/3(ErrSwitch)
  Demux/2 -> StErrSet_Wave/4(StWaveErrAmp)

== system GS_model/Subsystem2/Subsystem/Sensor/StA&B&C&DModel1/StAMathModel2/StErrSet/Triggered Subsystem1 ==
  In1 : Inport
  Enable : EnablePort
  Out1 : Outport  InitialOutput=0
  wires:
  In1/1 -> Out1/1

== system GS_model/Subsystem2/Subsystem/Sensor/StA&B&C&DModel1/StAMathModel2/StErrSet/Triggered Subsystem2 ==
  In1 : Inport
  Enable : EnablePort
  Out1 : Outport
  wires:
  In1/1 -> Out1/1

== system GS_model/Subsystem2/Subsystem/Sensor/StA&B&C&DModel1/StAMathModel2/StErrSet/Triggered Subsystem3 ==
  In1 : Inport
  Enable : EnablePort
  Out1 : Outport
  wires:
  In1/1 -> Out1/1

== system GS_model/Subsystem2/Subsystem/Sensor/StA&B&C&DModel1/StAMathModel2/StErrSet/Triggered Subsystem4 ==
  In1 : Inport
  Enable : EnablePort
  Out1 : Outport
  wires:
  In1/1 -> Out1/1

== system GS_model/Subsystem2/Subsystem/Sensor/StA&B&C&DModel1/StAMathModel2/StErrSet/Triggered Subsystem5 ==
  In1 : Inport
  Enable : EnablePort
  Out1 : Outport  InitialOutput=0
  wires:
  In1/1 -> Out1/1

== system GS_model/Subsystem2/Subsystem/Sensor/StA&B&C&DModel1/StAMathModel2/StMathModel/3 ==
  TC_StNoiseCoff : Inport
  Cons_StNoise : Inport  Port=2
  Constant : Constant
  Demux : Demux
  Mux : Mux  Inputs=2
  Product : Product
  Quaternion Normalize : sharedutil/Quaternion Normalize  aMode=aMode
      settings: SourceProductBaseCode=AE,PW,MT,VE,VP
  VoltA1 : Scope  NumInputPorts=4
  theta/2 : Gain  Gain=0.5
  Q_StNoise : Outport
  wires:
  Mux/1 -> Quaternion Normalize/1, Demux/1
  Quaternion Normalize/1 -> Q_StNoise/1
  Constant/1 -> Mux/1
  Demux/2 -> VoltA1/2
  Demux/3 -> VoltA1/3
  Demux/4 -> VoltA1/4
  Demux/1 -> VoltA1/1
  Cons_StNoise/1 -> Product/1
  TC_StNoiseCoff/1 -> Product/2
  Product/1 -> theta/2/1
  theta/2/1 -> Mux/2

== system GS_model/Subsystem2/Subsystem/Sensor/StA&B&C&DModel1/StAMathModel2/StMathModel/Triggered Subsystem1 ==
  In1 : Inport
  Enable : EnablePort
  Out1 : Outport  InitialOutput=[1;0;0;0]
  wires:
  In1/1 -> Out1/1

== system GS_model/Subsystem2/Subsystem/Sensor/StA&B&C&DModel1/StAMathModel2/StMathModel/Triggered Subsystem2 ==
  In1 : Inport
  Enable : EnablePort
  Out1 : Outport  InitialOutput=1
  wires:
  In1/1 -> Out1/1

== system GS_model/Subsystem2/Subsystem/Sensor/StA&B&C&DModel1/StAMathModel2/Subsystem/Subsystem ==
  note: Qbs
  Sun_b : Inport
  Sunshine : Inport  Port=2
  Qsb_StAFix : Inport  Port=3
  SEA : Inport  Port=4
  EEA : Inport  Port=5
  Qob : Inport  Port=6
  Acos : Trigonometry  Operator=acos
  Acos1 : Trigonometry  Operator=acos
  Compare To Constant : simulink/Logic and Bit Operations/Compare To Constant  relop===  const=1  OutDataTypeStr=boolean
  Constant : Constant  Value=St_SightAxis
  Constant1 : Constant  Value=[0;0;1]
  Constant3 : Constant  Value=St_EarthAtomAgl
  Cos : Trigonometry  Operator=cos
  Cos1 : Trigonometry  Operator=cos
  Data Type Conversion : DataTypeConversion  OutDataTypeStr=double
  Logical Operator : Logic  AllPortsSameDT=off  OutDataTypeStr=boolean
  Logical Operator1 : Logic  Operator=OR  AllPortsSameDT=off  OutDataTypeStr=boolean
  Logical Operator2 : Logic  Operator=NOT  AllPortsSameDT=off  OutDataTypeStr=boolean
  MatrixMultiply{,1..4} (5 alike) : Product  Multiplication=Matrix(*)
  Mux : Mux  Inputs=2
  Quaternion Inverse : aerolibutil/Quaternion Inverse
  Quaternions to Direction Cosine Matrix : sharedtransform/Quaternions to  Direction Cosine Matrix  aMode=aMode
      settings: SourceProductBaseCode=AE,PW,MT,VE,VP
  Quaternions to Direction Cosine Matrix1 : sharedtransform/Quaternions to  Direction Cosine Matrix  aMode=aMode
      settings: SourceProductBaseCode=AE,PW,MT,VE,VP
  Relational Operator : RelationalOperator  OutDataTypeStr=boolean  RndMeth=Simplest
  Relational Operator1 : RelationalOperator  OutDataTypeStr=boolean  RndMeth=Simplest
  Sum : Sum  Inputs=|++
  Transpose : Math  Operator=transpose  SaturateOnIntegerOverflow=on
  Valid : Outport
  Agl_St&SunEarth : Outport  Port=2
  wires:
  Transpose/1 -> MatrixMultiply4/1, MatrixMultiply1/1
  Constant3/1 -> Sum/2
  Logical Operator/1 -> Logical Operator1/1
  Cos/1 -> Relational Operator/2
  Quaternions to Direction Cosine Matrix1/1 -> MatrixMultiply2/1
  SEA/1 -> Cos/1
  Qob/1 -> Quaternions to Direction Cosine Matrix1/1
  MatrixMultiply3/1 -> MatrixMultiply4/2
  Qsb_StAFix/1 -> Quaternion Inverse/1
  Quaternions to Direction Cosine Matrix/1 -> MatrixMultiply3/1, MatrixMultiply/1
  Sun_b/1 -> MatrixMultiply/2
  Constant1/1 -> MatrixMultiply2/2
  MatrixMultiply2/1 -> MatrixMultiply3/2
  Cos1/1 -> Relational Operator1/2
  Quaternion Inverse/1 -> Quaternions to Direction Cosine Matrix/1
  Relational Operator/1 -> Logical Operator/2
  Constant/1 -> Transpose/1
  MatrixMultiply4/1 -> Acos1/1, Relational Operator1/1
  Sunshine/1 -> Compare To Constant/1
  EEA/1 -> Sum/1
  Relational Operator1/1 -> Logical Operator1/2
  Acos/1 -> Mux/1
  Acos1/1 -> Mux/2
  Sum/1 -> Cos1/1
  MatrixMultiply1/1 -> Relational Operator/1, Acos/1
  Compare To Constant/1 -> Logical Operator/1
  MatrixMultiply/1 -> MatrixMultiply1/2
  Mux/1 -> Agl_St&SunEarth/1
  Logical Operator2/1 -> Data Type Conversion/1
  Data Type Conversion/1 -> Valid/1
  Logical Operator1/1 -> Logical Operator2/1

== system GS_model/Subsystem2/Subsystem/Sensor/StA&B&C&DModel1/StAMathModel2/Subsystem/Triggered Subsystem2 ==
  In1 : Inport
  Enable : EnablePort
  Out1 : Outport  InitialOutput=1
  wires:
  In1/1 -> Out1/1

== system GS_model/Subsystem2/Subsystem/Sensor/StA&B&C&DModel1/StAMathModel3/StErrSet/From Q to W ==
  q : Inport
  Acos : Trigonometry  Operator=acos
  Delay : Delay  DelayLength=1
  Demux6 : Demux  Outputs=[1;3]
  Gain : Gain  Gain=2/T_Simu
  Normalize Vector : vrlib/Utilities/Normalize Vector  maxzero=0
  Product : Product
  Product1 : Product
  Quaternion Division : aerolibutil/Quaternion Division
      settings: SourceProductBaseCode=AE
  Selector : Selector  InputPortWidth=4  IndexOptions=Index vector (dialog)  Indices=1  OutputSizes=1
  Sign : Signum
  w : Outport
  wires:
  Product1/1 -> Demux6/1
  Sign/1 -> Product1/1
  Quaternion Division/1 -> Product1/2, Selector/1
  Selector/1 -> Sign/1
  Delay/1 -> Quaternion Division/2
  Normalize Vector/1 -> Product/2
  Product/1 -> w/1
  Demux6/2 -> Normalize Vector/1
  q/1 -> Quaternion Division/1, Delay/1
  Gain/1 -> Product/1
  Demux6/1 -> Acos/1
  Acos/1 -> Gain/1

== system GS_model/Subsystem2/Subsystem/Sensor/StA&B&C&DModel1/StAMathModel3/StErrSet/If Action Subsystem ==
  In1 : Inport
  Action Port : ActionPort  ActionType=then
  Out1 : Outport
  wires:
  In1/1 -> Out1/1

== system GS_model/Subsystem2/Subsystem/Sensor/StA&B&C&DModel1/StAMathModel3/StErrSet/If Action Subsystem1 ==
  In1 : Inport
  Action Port : ActionPort  ActionType=else
  Out1 : Outport
  wires:
  In1/1 -> Out1/1

== system GS_model/Subsystem2/Subsystem/Sensor/StA&B&C&DModel1/StAMathModel3/StErrSet/StAErrSet ==
  note: Amp
  note: Switch
  note: AmpCoff
  note: Period
  note: Switch
  Qis_St : Inport
  TC_StErr_Constant : Inport  Port=2
  TC_StErr_WildValue : Inport  Port=3
  TC_StErr_Jump : Inport  Port=4
  TC_StErr_Wave : Inport  Port=5
  AssErrSet_WildValue : Subsystem
  Demux : Demux  Outputs=2
  Demux1 : Demux  Outputs=3
  JumpSet : Constant  Value=[0;6/180*pi;0]
  StErrSet_Constant : Subsystem
  StErrSet_Jump : Subsystem
  StErrSet_Wave : Subsystem
  Terminator : Terminator
  WaveSet : SignalGenerator  WaveForm=square  Amplitude=1/180*pi
  WildValueSet : Constant  Value=1.2
  TM_St_Qis : Outport
  wires:
  Demux/2 -> StErrSet_Wave/4(StWaveErrAmp)
  Demux/1 -> StErrSet_Wave/3(ErrSwitch)
  WaveSet/1 -> StErrSet_Wave/2(ErrValue)
  StErrSet_Wave/1(Q_out) -> TM_St_Qis/1
  StErrSet_Jump/1(Q_out) -> StErrSet_Wave/1(Qin)
  Demux1/3 -> StErrSet_Jump/4(StJumpErrAmpCoff)
  Demux1/1 -> StErrSet_Jump/3(ErrSwitch)
  TC_StErr_Jump/1 -> Demux1/1
  Demux1/2 -> Terminator/1
  JumpSet/1 -> StErrSet_Jump/2(ErrValue)
  AssErrSet_WildValue/1(Q_out) -> StErrSet_Jump/1(Qin)
  WildValueSet/1 -> AssErrSet_WildValue/2(ErrValue)
  TC_StErr_WildValue/1 -> AssErrSet_WildValue/3(ErrSwitch)
  StErrSet_Constant/1(Q_out) -> AssErrSet_WildValue/1(Qin)
  TC_StErr_Constant/1 -> StErrSet_Constant/2(ErrSwitch)
  Qis_St/1 -> StErrSet_Constant/1(Q_in)
  TC_StErr_Wave/1 -> Demux/1

== system GS_model/Subsystem2/Subsystem/Sensor/StA&B&C&DModel1/StAMathModel3/StErrSet/Triggered Subsystem1 ==
  In1 : Inport
  Enable : EnablePort
  Out1 : Outport  InitialOutput=0
  wires:
  In1/1 -> Out1/1

== system GS_model/Subsystem2/Subsystem/Sensor/StA&B&C&DModel1/StAMathModel3/StErrSet/Triggered Subsystem2 ==
  In1 : Inport
  Enable : EnablePort
  Out1 : Outport
  wires:
  In1/1 -> Out1/1

== system GS_model/Subsystem2/Subsystem/Sensor/StA&B&C&DModel1/StAMathModel3/StErrSet/Triggered Subsystem3 ==
  In1 : Inport
  Enable : EnablePort
  Out1 : Outport
  wires:
  In1/1 -> Out1/1

== system GS_model/Subsystem2/Subsystem/Sensor/StA&B&C&DModel1/StAMathModel3/StErrSet/Triggered Subsystem4 ==
  In1 : Inport
  Enable : EnablePort
  Out1 : Outport
  wires:
  In1/1 -> Out1/1

== system GS_model/Subsystem2/Subsystem/Sensor/StA&B&C&DModel1/StAMathModel3/StErrSet/Triggered Subsystem5 ==
  In1 : Inport
  Enable : EnablePort
  Out1 : Outport  InitialOutput=0
  wires:
  In1/1 -> Out1/1

== system GS_model/Subsystem2/Subsystem/Sensor/StA&B&C&DModel1/StAMathModel3/StMathModel/3 ==
  TC_StNoiseCoff : Inport
  Cons_StNoise : Inport  Port=2
  Constant : Constant
  Demux : Demux
  Mux : Mux  Inputs=2
  Product : Product
  Quaternion Normalize : sharedutil/Quaternion Normalize  aMode=aMode
      settings: SourceProductBaseCode=AE,PW,MT,VE,VP
  VoltA1 : Scope  NumInputPorts=4
  theta/2 : Gain  Gain=0.5
  Q_StNoise : Outport
  wires:
  theta/2/1 -> Mux/2
  Product/1 -> theta/2/1
  TC_StNoiseCoff/1 -> Product/2
  Cons_StNoise/1 -> Product/1
  Demux/1 -> VoltA1/1
  Demux/4 -> VoltA1/4
  Demux/3 -> VoltA1/3
  Demux/2 -> VoltA1/2
  Constant/1 -> Mux/1
  Quaternion Normalize/1 -> Q_StNoise/1
  Mux/1 -> Demux/1, Quaternion Normalize/1

== system GS_model/Subsystem2/Subsystem/Sensor/StA&B&C&DModel1/StAMathModel3/StMathModel/Triggered Subsystem1 ==
  In1 : Inport
  Enable : EnablePort
  Out1 : Outport  InitialOutput=[1;0;0;0]
  wires:
  In1/1 -> Out1/1

== system GS_model/Subsystem2/Subsystem/Sensor/StA&B&C&DModel1/StAMathModel3/StMathModel/Triggered Subsystem2 ==
  In1 : Inport
  Enable : EnablePort
  Out1 : Outport  InitialOutput=1
  wires:
  In1/1 -> Out1/1
